simulink model "testBCIRobot3f_sim"  (Simulink 7.4)
settings: Solver=FixedStepDiscrete  SolverMode=SingleTasking  StartTime=0.0  StopTime=10  FixedStep=0.002  MaxStep=0.02  RelTol=1e-3  AbsTol=1e-6
libraries: simulink_extras x2
CloseFcn:
  | rtwprivate ssgencode ModelCloseRequest MC_AD
settings Model: Creator=fwornle  LastModifiedBy=fw  ExtModeTrigDuration=5000  ExtModeLogAll=off
settings ConfigSet: Description=rtmc9s12target_R2008a
settings DataIOCC: LimitDataPoints=off  SaveOutput=off  SaveTime=off  SignalLoggingName=sigsOut
settings OptimizationCC: BlockReduction=off  BooleanDataType=off  InitFltsAndDblsToZero=on
settings DebuggingCC: SaveWithParameterizedLinksMsg=none  SignalResolutionControl=TryResolveAllWithWarning  SolverPrmCheckMsg=none  MultiTaskDSMMsg=warning  MultiTaskCondExecSysMsg=none  StrictBusMsg=None
settings HardwareCC: ProdBitPerInt=16  ProdEndianess=BigEndian  ProdWordSize=16  ProdHWDeviceType=Motorola HC12  TargetHWDeviceType=32-bit Generic  ProdEqTarget=off
settings RTWCC: GenerateMakefile=off  TemplateMakefile=grt_msvc.tmf  Description="Visual C/C++ Project Makefile only for the \"grt\" target"  ProcessScript=grt_make_rtw_hook  IncludeERTFirstTime=on
settings GRTTargetCC: TargetFcnLib=ansi_tfl_tmw.mat

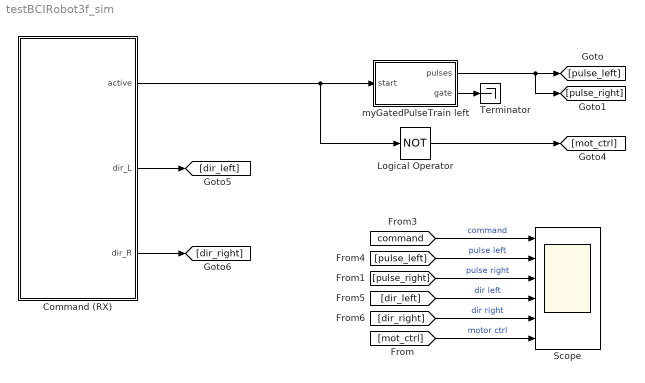
== system testBCIRobot3f_sim ==
  Command (RX) : Subsystem
  Logical Operator : Logic  Operator=NOT  AllPortsSameDT=off
  Scope : Scope  NumInputPorts=6
      settings: TimeRange=10  YMin=-1~-5~-5~-5~-5~-5  YMax=4~5~5~5~5~5
  Terminator : Terminator
  myGatedPulseTrain left : Subsystem  mask{Tcount=0.02, Nsamp=30}
      mask prompts: Tcount "Sample time"; Nsamp "Number of samples"
      mask init:
      | % each period has an on-phase and an off-phase
      | Ncount = 2*Nsamp;
  wires:
  Logical Operator/1 -> [mot_ctrl]
  myGatedPulseTrain left/2(gate) -> Terminator/1
  myGatedPulseTrain left/1(pulses) -> [pulse_left], [pulse_right]
  Command (RX)/1(active) -> myGatedPulseTrain left/1(start), Logical Operator/1
  Command (RX)/2(dir_L) -> [dir_left]
  Command (RX)/3(dir_R) -> [dir_right]
  [command] -> Scope/1  "command"
  [pulse_left] -> Scope/2  "pulse left"
  [pulse_right] -> Scope/3  "pulse right"
  [dir_left] -> Scope/4  "dir left"
  [dir_right] -> Scope/5  "dir right"
  [mot_ctrl] -> Scope/6  "motor ctrl"

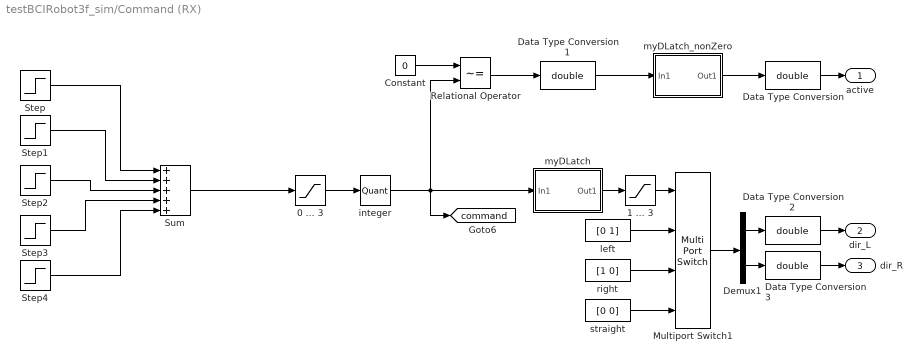
== system testBCIRobot3f_sim/Command (RX) ==
  " left " : Constant  Value=[0 1]  OutDataTypeMode=double  OutDataType=sfix(16)  OutScaling=2^0  OutDataTypeStr=double
  " right " : Constant  Value=[1 0]  OutDataTypeMode=double  OutDataType=sfix(16)  OutScaling=2^0  OutDataTypeStr=double
  " straight " : Constant  Value=[0 0]  OutDataTypeMode=double  OutDataType=sfix(16)  OutScaling=2^0  OutDataTypeStr=double
  0 ... 3 : Saturate  UpperLimit=3  LowerLimit=0  SampleTime=0.002
  1 ... 3 : Saturate  UpperLimit=3  LowerLimit=1
  Constant : Constant  Value=0  OutDataType=sfix(16)  OutScaling=2^0
  Data Type Conversion{,1..3} (4 alike) : DataTypeConversion  OutDataTypeMode=double  OutDataType=sfix(16)  OutScaling=2^0  OutDataTypeStr=double  SaturateOnIntegerOverflow=on  RndMeth=Zero
  Demux1 : Demux  Outputs=2
  Multiport Switch1 : MultiPortSwitch  SaturateOnIntegerOverflow=on
  Relational Operator : RelationalOperator  Operator=~=  LogicOutDataTypeMode=Specify via dialog  OutDataTypeStr=uint(8)
  Step : Step  After=3  SampleTime=0
  Step1 : Step  Time=2  After=-2  SampleTime=0
  Step2 : Step  Time=2.1  After=-1  SampleTime=0
  Step3 : Step  Time=4  After=2  SampleTime=0
  Step4 : Step  Time=4.2  After=-2  SampleTime=0
  Sum : Sum  Inputs=+++++  OutDataType=sfix(16)  OutScaling=2^0  SaturateOnIntegerOverflow=on
  integer : Quantizer  QuantizationInterval=1
  myDLatch : Subsystem
  myDLatch_nonZero : Subsystem
  active : Outport  OutDataType=sfix(16)  OutScaling=2^0
  dir_L : Outport  Port=2  OutDataType=sfix(16)  OutScaling=2^0
  dir_R : Outport  Port=3  OutDataType=sfix(16)  OutScaling=2^0
  tag scope: command=global
  wires:
  0 ... 3/1 -> integer/1
  " left "/1 -> Multiport Switch1/2
  " right "/1 -> Multiport Switch1/3
  " straight "/1 -> Multiport Switch1/4
  Multiport Switch1/1 -> Demux1/1
  Demux1/1 -> Data Type Conversion2/1
  Demux1/2 -> Data Type Conversion3/1
  1 ... 3/1 -> Multiport Switch1/1
  Data Type Conversion2/1 -> dir_L/1
  Data Type Conversion3/1 -> dir_R/1
  Constant/1 -> Relational Operator/1
  Relational Operator/1 -> Data Type Conversion1/1
  Data Type Conversion/1 -> active/1
  myDLatch/1(Out1) -> 1 ... 3/1
  Sum/1 -> 0 ... 3/1
  integer/1 -> myDLatch/1(In1), Relational Operator/2, [command]
  Step/1 -> Sum/1
  Step1/1 -> Sum/2
  Step2/1 -> Sum/3
  Step3/1 -> Sum/4
  Step4/1 -> Sum/5
  myDLatch_nonZero/1(Out1) -> Data Type Conversion/1
  Data Type Conversion1/1 -> myDLatch_nonZero/1(In1)

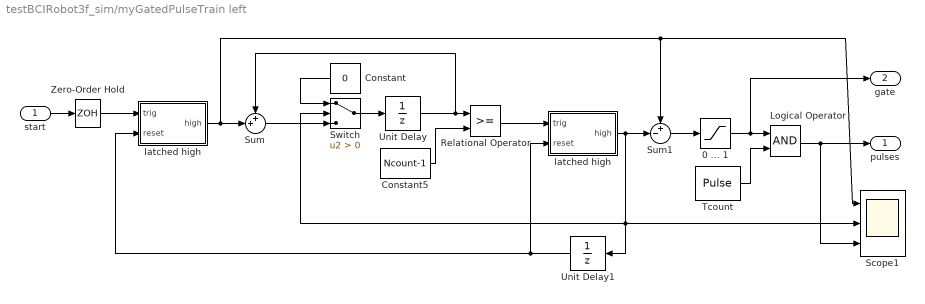
== system testBCIRobot3f_sim/myGatedPulseTrain left ==
  start : Inport  OutDataType=sfix(16)  OutScaling=2^0
  " latched high " : Subsystem
  0 ... 1 : Saturate  UpperLimit=1  LowerLimit=0
  Constant : Constant  Value=0  OutDataType=sfix(16)  OutScaling=2^0
  Constant5 : Constant  Value=Ncount-1  OutDataType=sfix(16)  OutScaling=2^0
  Logical Operator : Logic  AllPortsSameDT=off
  Relational Operator : RelationalOperator  LogicOutDataTypeMode=Specify via dialog  OutDataTypeStr=uint(8)
  Scope1 : Scope  NumInputPorts=3
      settings: YMin=-5~-5~-5  YMax=5~5~5
  Sum : Sum  Inputs=++|  OutDataType=sfix(16)  OutScaling=2^0
  Sum1 : Sum  Inputs=+-|  OutDataType=sfix(16)  OutScaling=2^0
  Switch : Switch  Criteria=u2 > Threshold
  Tcount : DiscretePulseGenerator  Amplitude=1  Period=2  PulseWidth=1  PhaseDelay=0  SampleTime=Tcount
  Unit Delay : UnitDelay  SampleTime=Tcount
  Unit Delay1 : UnitDelay  SampleTime=Tcount
  Zero-Order Hold : ZeroOrderHold  SampleTime=Tcount
  latched high : Subsystem
  pulses : Outport  OutDataType=sfix(16)  OutScaling=2^0
  gate : Outport  Port=2  OutDataType=sfix(16)  OutScaling=2^0
  wires:
  Zero-Order Hold/1 -> latched high/1(trig)
  Logical Operator/1 -> Scope1/3, pulses/1
  Tcount/1 -> Logical Operator/2
  0 ... 1/1 -> gate/1, Logical Operator/1
  Unit Delay1/1 -> latched high/2(reset), " latched high "/2(reset)
  " latched high "/1(high) -> Unit Delay1/1, Switch/2, Scope1/2, Sum1/2
  Relational Operator/1 -> " latched high "/1(trig)
  Sum1/1 -> 0 ... 1/1
  Switch/1 -> Unit Delay/1
  Unit Delay/1 -> Sum/1, Relational Operator/1
  Sum/1 -> Switch/3
  Constant/1 -> Switch/1
  Constant5/1 -> Relational Operator/2
  start/1 -> Zero-Order Hold/1
  latched high/1(high) -> Scope1/1, Sum1/1, Sum/2

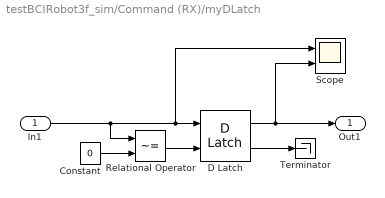
== system testBCIRobot3f_sim/Command (RX)/myDLatch ==
  In1 : Inport  OutDataType=sfix(16)  OutScaling=2^0
  Constant : Constant  Value=0  OutDataType=sfix(16)  OutScaling=2^0
  D Latch : simulink_extras/Flip Flops/D Latch  SystemSampleTime=-1
  Relational Operator : RelationalOperator  Operator=~=
  Scope : Scope  NumInputPorts=2
      settings: YMin=-5~-5  YMax=5~5  SaveName=ScopeData3
  Terminator : Terminator
  Out1 : Outport  OutDataType=sfix(16)  OutScaling=2^0
  wires:
  D Latch/2 -> Terminator/1
  D Latch/1 -> Out1/1, Scope/2
  In1/1 -> Relational Operator/1, D Latch/1, Scope/1
  Constant/1 -> Relational Operator/2
  Relational Operator/1 -> D Latch/2

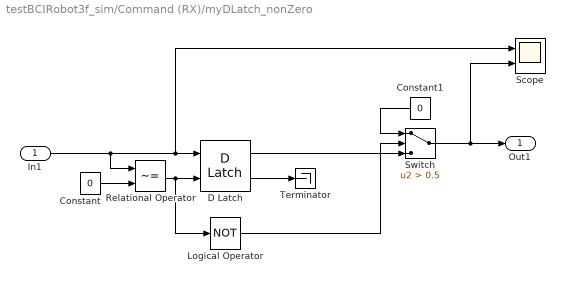
== system testBCIRobot3f_sim/Command (RX)/myDLatch_nonZero ==
  In1 : Inport  OutDataType=sfix(16)  OutScaling=2^0
  Constant : Constant  Value=0  OutDataType=sfix(16)  OutScaling=2^0
  Constant1 : Constant  Value=0  OutDataType=sfix(16)  OutScaling=2^0
  D Latch : simulink_extras/Flip Flops/D Latch  SystemSampleTime=-1
  Logical Operator : Logic  Operator=NOT  AllPortsSameDT=off
  Relational Operator : RelationalOperator  Operator=~=
  Scope : Scope  NumInputPorts=2
      settings: YMin=-5~-5  YMax=5~5  SaveName=ScopeData3
  Switch : Switch  Criteria=u2 > Threshold  Threshold=0.5  SaturateOnIntegerOverflow=on
  Terminator : Terminator
  Out1 : Outport  OutDataType=sfix(16)  OutScaling=2^0
  wires:
  Relational Operator/1 -> D Latch/2, Logical Operator/1
  Constant/1 -> Relational Operator/2
  In1/1 -> Scope/1, D Latch/1, Relational Operator/1
  D Latch/1 -> Switch/3
  D Latch/2 -> Terminator/1
  Switch/1 -> Out1/1, Scope/2
  Constant1/1 -> Switch/1
  Logical Operator/1 -> Switch/2

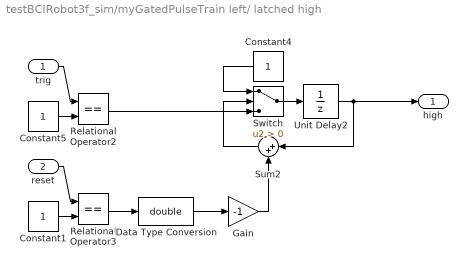
== system testBCIRobot3f_sim/myGatedPulseTrain left/ latched high  ==
  trig : Inport  OutDataType=sfix(16)  OutScaling=2^0
  reset : Inport  Port=2  OutDataType=sfix(16)  OutScaling=2^0
  Constant1 : Constant  OutDataType=sfix(16)  OutScaling=2^0
  Constant4 : Constant  OutDataType=sfix(16)  OutScaling=2^0
  Constant5 : Constant  OutDataType=sfix(16)  OutScaling=2^0
  Data Type Conversion : DataTypeConversion  OutDataTypeMode=double  OutDataType=sfix(16)  OutScaling=2^0  OutDataTypeStr=double  SaturateOnIntegerOverflow=on  RndMeth=Zero
  Gain : Gain  Gain=-1  ParameterDataType=sfix(16)  ParameterScaling=2^0  OutDataType=sfix(16)  OutScaling=2^0  SaturateOnIntegerOverflow=on  OutDataTypeStr=Inherit: Same as input  ParamDataTypeStr=Inherit: Same as input
  Relational Operator2 : RelationalOperator  Operator===  LogicOutDataTypeMode=Specify via dialog  OutDataTypeStr=uint(8)
  Relational Operator3 : RelationalOperator  Operator===  LogicOutDataTypeMode=Specify via dialog  OutDataTypeStr=uint(8)
  Sum2 : Sum  Inputs=|++  OutDataType=sfix(16)  OutScaling=2^0
  Switch : Switch  Criteria=u2 > Threshold
  Unit Delay2 : UnitDelay  SampleTime=-1
  high : Outport  OutDataType=sfix(16)  OutScaling=2^0
  wires:
  trig/1 -> Relational Operator2/1
  reset/1 -> Relational Operator3/1
  Data Type Conversion/1 -> Gain/1
  Gain/1 -> Sum2/2
  Relational Operator3/1 -> Data Type Conversion/1
  Constant1/1 -> Relational Operator3/2
  Sum2/1 -> Switch/2
  Switch/1 -> Unit Delay2/1
  Constant4/1 -> Switch/1
  Unit Delay2/1 -> high/1, Sum2/1
  Relational Operator2/1 -> Switch/3
  Constant5/1 -> Relational Operator2/2

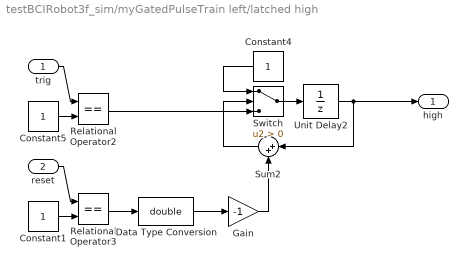
== system testBCIRobot3f_sim/myGatedPulseTrain left/latched high ==
  trig : Inport  OutDataType=sfix(16)  OutScaling=2^0
  reset : Inport  Port=2  OutDataType=sfix(16)  OutScaling=2^0
  Constant1 : Constant  OutDataType=sfix(16)  OutScaling=2^0
  Constant4 : Constant  OutDataType=sfix(16)  OutScaling=2^0
  Constant5 : Constant  OutDataType=sfix(16)  OutScaling=2^0
  Data Type Conversion : DataTypeConversion  OutDataTypeMode=double  OutDataType=sfix(16)  OutScaling=2^0  OutDataTypeStr=double  SaturateOnIntegerOverflow=on  RndMeth=Zero
  Gain : Gain  Gain=-1  ParameterDataType=sfix(16)  ParameterScaling=2^0  OutDataType=sfix(16)  OutScaling=2^0  SaturateOnIntegerOverflow=on  OutDataTypeStr=Inherit: Same as input  ParamDataTypeStr=Inherit: Same as input
  Relational Operator2 : RelationalOperator  Operator===  LogicOutDataTypeMode=Specify via dialog  OutDataTypeStr=uint(8)
  Relational Operator3 : RelationalOperator  Operator===  LogicOutDataTypeMode=Specify via dialog  OutDataTypeStr=uint(8)
  Sum2 : Sum  Inputs=|++  OutDataType=sfix(16)  OutScaling=2^0
  Switch : Switch  Criteria=u2 > Threshold
  Unit Delay2 : UnitDelay  SampleTime=-1
  high : Outport  OutDataType=sfix(16)  OutScaling=2^0
  wires:
  Constant5/1 -> Relational Operator2/2
  Relational Operator2/1 -> Switch/3
  Unit Delay2/1 -> Sum2/1, high/1
  Constant4/1 -> Switch/1
  Switch/1 -> Unit Delay2/1
  Sum2/1 -> Switch/2
  Constant1/1 -> Relational Operator3/2
  Relational Operator3/1 -> Data Type Conversion/1
  Gain/1 -> Sum2/2
  Data Type Conversion/1 -> Gain/1
  reset/1 -> Relational Operator3/1
  trig/1 -> Relational Operator2/1
